simulink model "dspafxr"  (Simulink 6.0)
settings: Solver=FixedStepDiscrete  SolverMode=SingleTasking  StartTime=0.0  StopTime=2  RelTol=1e-3  AbsTol=1e-6
PreLoadFcn:
  | load dspafxr;
undefined symbols (not defined in the file or in its folder): fs_afxr
libraries: dspsigops x1, dspsrcs4 x1
settings Model: Creator=don  LastModifiedBy=mkhan  ExtModeTrigMode=oneshot  ExtModeArmWhenConnect=off  SaveTime=off  SaveOutput=off  LimitDataPoints=off  SignalLoggingName=logsOut  IntegerOverflowMsg=none  BlockReductionOpt=off  ZeroCrossControl=UseLocalSettings  ProdHWDeviceType=Microprocessor  TargetHWChar=2  TargetHWWordLengths=8,16,32,32  RTWMathFcnLibMatFile=iso_c_tmw.mat  RTWOptions="-aEnforceIntegerDowncast=1 -aFoldNonRolledExpr=1 -aInlineInvariantSignals=1 -aInlineParameters=0 -aLocalBlockOutputs=1 -aRollThreshold=2 -aGenerateReport=0 -aGenCodeOnly=0 -aRTWVerbose=1 -aForceParamTrailComments=0 -aGenerateComments=1 -aIgnoreCustomStorageClasses=1 -aIncHierarchyInIds=0 -aMaxRTWIdLen=31 -aShowEliminatedStatements=0 -aPrefixModelToSubsysFcnNames=1 -aIncDataTypeInIds=0 -aInlinedPrmAccess=\"Literals\" -aTargetFcnLib=\"iso_c_tmw.mat\" -aGenerateFullHeader=1 -aIsPILTarget=0 -aExtMode=0 -aExtModeStaticAlloc=0 -aExtModeTesting=0 -aExtModeStaticAllocSize=1000000 -aExtModeTransport=0 -aLogVarNameModifier=\"rt_\" -aRTWCAPISignals=0 -aRTWCAPIParams=0"
settings DataIOCC: LimitDataPoints=off  SaveOutput=off  SaveTime=off  SignalLoggingName=logsOut
settings OptimizationCC: BlockReduction=off  BooleanDataType=off  MultiInstanced=off  RollThreshold=2
settings FormatCC: IgnoreBidirectionalLines=off
settings DebuggingCC: IntegerOverflowMsg=none
settings HardwareCC: ProdHWDeviceType=Microprocessor  ShiftRightIntArith=on  TargetHWCharacteristics=InheritFromRTWHook
settings CodeAppCC: FileBanners=off
settings GRTTargetCC: TargetFcnLib=iso_c_tmw.mat  IsERTTarget=off

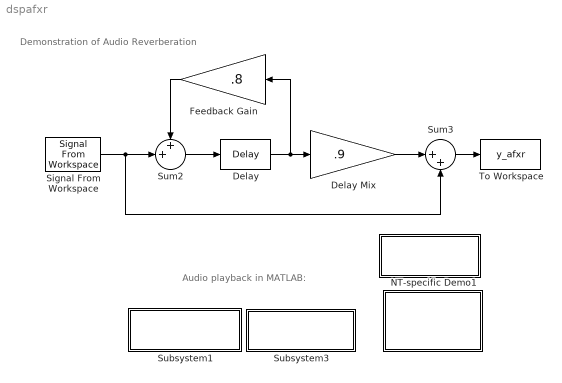
== system dspafxr ==
  note: Audio playback in MATLAB:
  note: Demonstration of
      | Audio Reverberation
  "  " : Subsystem
      mask Type: Frame-Based Simulation Info
      mask Display: disp('Info')
  Delay : dspsigops/Delay  dly_unit=Samples  delay=1800  ic_detail=on  dif_ic_for_ch=off  dif_ic_for_dly=off  ic=0  reset_popup=None
  Delay Mix : Gain  Gain=.9  SaturateOnIntegerOverflow=on
  Feedback Gain : Gain  Orientation=left  Gain=.8  SaturateOnIntegerOverflow=on
  NT-specific Demo1 : Subsystem
      settings: OpenFcn=dspafxr_win32
      mask Type: NT-only Demo
      mask Display: disp('PC/Windows\nDemo')
  Signal From Workspace : dspsrcs4/Signal From Workspace  X=x_afxr  Ts=1/fs_afxr  nsamps=128  OutputAfterFinalValue=Setting to zero
  Subsystem1 : Subsystem
      settings: OpenFcn=if exist('x_afxr','var') & exist('fs_afxr','var'), sound(x_afxr,fs_afxr); else errordlg('Data not found in workspace - reload demo model.','Signal Processing Blockset Demo Error'); end
      mask Display: disp('Original\nSignal')
  Subsystem3 : Subsystem
      settings: OpenFcn=if exist('y_afxr','var') & exist('fs_afxr','var'), sound(y_afxr,fs_afxr); else errordlg('You must run the simulation first.','Signal Processing Blockset Demo Error'); end
      mask Display: disp('Enhanced\nSignal')
  Sum2 : Sum  Inputs=++|  SaturateOnIntegerOverflow=on  InputSameDT=on
  Sum3 : Sum  Inputs=|++  SaturateOnIntegerOverflow=on  InputSameDT=on
  To Workspace : ToWorkspace  VariableName=y_afxr  SampleTime=-1  SaveFormat=Array
  wires:
  Sum3/1 -> To Workspace/1
  Signal From Workspace/1 -> Sum2/2, Sum3/2
  Sum2/1 -> Delay/1
  Feedback Gain/1 -> Sum2/1
  Delay/1 -> Delay Mix/1, Feedback Gain/1
  Delay Mix/1 -> Sum3/1

== system dspafxr/   ==
  note: This simulation of audio reverberation
      | employs frame-based processing.
      |
      | By default, the simulation uses
      | 128 samples per frame.

== system dspafxr/NT-specific Demo1 ==

== system dspafxr/Subsystem1 ==

== system dspafxr/Subsystem3 ==
